simulink model "BiT_Template_V4"  (R2025b)
settings: Solver=FixedStepAuto  StartTime=0.0  StopTime=90  FixedStep=0.005  RelTol=1e-3
StopFcn:
  | user_confirmed = true;
  | disp('Gestoppt?!')
  | 
  | % stop(t);
  | % delete(t);
  | 
  | %% Switch to Config Mode
  | %Tc3_AI.sysManager.ActivateConfiguration();
  | %
  | % Tc3_AI.SwitchToConfig('local')
  | %
  | % %save Solution
  | % Tc3_AI.SaveSolution();
  | %
  | % %% Close Aktive VS Instance
  | % Tc3_AI.closeVsInstance();
libraries: simulink x1, slpidlib x1
settings Model: SimulationMode=external  Creator=clemensm  LastModifiedBy=Felix
settings OptimizationCC: LocalBlockOutputs=off
settings RTWCC: SystemTargetFile=TwinCatGrt.tlc  GenCodeOnly=on  GenerateMakefile=off  TemplateMakefile=tcgrt_msbuild.tmf  TargetLang=C++  Description=TwinCAT GRT Target
settings STFCustomTargetCC: SystemTargetFile=TwinCatGrt.tlc  TargetLangStandard=C++11 (ISO)  CombineOutputUpdateFcns=on  CodeInterfacePackaging=Reusable function  CPPClassGenCompliant=on  GRTInterface=off  GenerateAllocFcn=on  TcCom_OnlineChange=off  TcProject_PublishTcRTx64=on  TcProject_PublishConfiguration=Release  TcProject_CppLanguageStandard=Default  TcProject_Description=TwinCAT executable file, generated by TwinCAT $<ModuleGenerator:ProductId>  TcCom_GroupName=TE140x|Simulink Modules  TcProject_DataExchangeModulesVersion=$<ModuleGenerator:DataExchange:Version>  TcCom_BlockDiagramDebugInfoExport=on  TcCom_OutputDataAccess=Output Source DataArea  TcCom_OutputCreateSymbols=on  TcProject_LibraryCategories=$<VendorName>  TcCom_DWorkCreateSymbols=on  TcProject_UseStaticStlString=off  TcProject_PlcVarPrefixes=PVOID=p | BOOL=b | BOOL32=b | DATE=d | TIME_OF_DATE=td | TIME=t | LTIME=t | GUID=n  TcCom_UpdateExceptionHandling=CallerExceptions  TcCom_VariableSymbolMapping=Identical  TcProject_Publish=on  TcCom_BlockIoReadOnly=on  TcProject_VendorName=TE140x Module Vendor  TcCom_InputInitValues=off  TcCom_InputDataAccess=Input Destination DataArea  TcProject_LowestCompatibleTcBuild=$<TwinCAT:Version:BUILD>  TcProject_SignTwinCatCertName=MCI_2024_OEM.tccert  TcCom_StepSizeAdaptation=RequireMatchingTaskCycleTime  TcCom_OemLicenses=$<Project:OemLicenses>  TcCom_ExecutionSequence=UpdateBeforeOutputMapping  TcCom_OriginalIoBlockNames=off  TcProject_BuildWithWdk=inherit default  TcProject_GeneratePlcLibrary=off  TcProject_ForceRebuildForPublish=off  TcCom_CallerVerification=Default  TcProject_PublishTcRTx86=on  TcCom_TcComWrapperFbProperties=off  TcProject_StaticStlStringCapacity=Auto  TcCom_StrictAccessLock=on  TcProject_PublishTcOSARMv8A=off  TcProject_UseIntrinsics=on  TcProject_DrvProductVersion=$<DrvFileVersion>  TcProject_IncrementVersion=Revision  TcProject_VendorIcon=$<TE140x:Icon>  TcProject_PreferIntOverLong=off  TcProject_ClassFactoryName=$<Project:Name>  TcCom_ExtModeRtAllowForParameterChange=on  TcProject_InstallPlcLibrary=off  TcCom_BlockDiagramVariableAccess=AssignToParent  TcCom_OnlineChangeRestoreDataAreas=off  TcProject_UseTmxExtension=Auto  TcCom_ModuleCaller=CyclicTask  TcCom_InputReadOnly=off  TcCom_DWorkReadOnly=on  TcCom_BlockDiagramExport=on  TcProject_PublishTcOSx64=off  TcCom_ExtendSignalResolution=on  TcPlcFb_Generate=off  TcPlcFb_ExtModeRtAllowForParameterChange=off  TcProject_PublishPlatformtoolset=Auto  TcCom_ParametersCreateSymbols=on  TcProject_UseDataExchangeModules=off  TcProject_CreateScopedEnums=Auto  TcCom_GlobalParamDefaultSharing=Define  TcCom_ContStateCreateSymbols=on  TcPlcFb_MonitorExecutionTime=off  TcProject_UseCodeInfoExporter=on  TcCom_GroupDisplayName=$<GroupName>  TcCom_Generate=on  TcCom_InitExceptionHandling=CallerExceptions  TcProject_Copyright=Copyright $<VendorName> $<LocalDateTime:%Y>  TcCom_ResolveMaskedSubsystems=on  TcCom_ExtModeRtAllowExecutionCommands=on  TcPlcFb_ExtModeRtAllowExecutionCommands=off  TcProject_PublishTcOSARMv7A=off  TcCom_BlockIoDataAccess=Internal DataArea  TcProject_SignWithTwinCatCertificate=inherit default  TcCom_TcComWrapperFb=off  TcCom_OutputReadOnly=on  TcCom_AccessLockState=Auto  TcProject_DeployRestart=off  TcProject_UseCodeDescriptor=on  TcProject_EnableNewPlatforms=off  TcCom_Legacy_ModuleBuildInfoParam=on  TcCom_ModuleIcon=$<TE140x:Icon>  TcPlcFb_OemLicenses=$<Project:OemLicenses>  TcCom_InputCreateSymbols=on  TcProject_PreferToolArchitectureX64=on  TcProject_DrvFileVersion=$<VersionFromFile>  TcCom_MonitorExecutionTime=off  TcCom_ContStateDataAccess=Internal DataArea  TcCom_ContStateReadOnly=on  TcProject_GenerateStructDutsWithDefaultValues=Auto  TcProject_LibCatPath=$<Project:Dir>\$<Project:Name>.libcat.xml  TcCom_TcComWrapperFbPropertyMonitoring=NoMonitoring  TcProject_CLanguageStandard=Default  TcCom_ExtModeRtWaitForStart=off  TcProject_PublishParallel=on  TcProject_PublishTcUMx86=off  TcProject_UseNativeBlockDiagramExport=off  TcPlcFb_UpdateExceptionHandling=CallerExceptions  TcCom_DataStoreReadOnly=off  TcPlcFb_ExtModeRtWaitForStart=off  TcCom_GroupIcon=$<TE140x:Icon>  TcProject_PublishTcUMx64=off  TcProject_VersionSrc=$<LatestTMFile>  TcCom_ExecutionInfoOutput=off  TcCom_ExecutionInfoParam=on  TcProject_ProjectDir=C:\TwinCAT\3.1\CustomConfig\Modules\Ctrl_only  TcProject_BuildSystem=Auto  TcCom_ParametersInitValues=on  TcCom_ParametersReadOnly=off  TcCom_ParametersDataAccess=Internal DataArea  TcProject_MaxVisibleArrayElements=200U  TcProject_PublishTcOSARMv7M=off  TcCom_ExecuteModelCode=on  TcCom_DWorkDataAccess=Internal DataArea  TcProject_CoderCppNamespace=coder  TcProject_Generate=on  TcProject_Versioning=Versioned  TcProject_GenerateVsSolution=No  TcProject_Verbosity=Normal  TcProject_CreateUniqueEnumItemNames=off  TcCom_DataStoreDataAccess=None  TcCom_AllowDataAreaForSharedData=off  TcProject_ProductName=$<ModuleGenerator:ProductId> $<ModuleGenerator:Version:MAJOR.MINOR>  TcCom_DataStoreCreateSymbols=on  TcProject_UseDescriptorCodeType=on  TcPlcFb_InitExceptionHandling=CallerExceptions  TcProject_TmxInstall=on  TcCom_BlockIoCreateSymbols=on
settings GRTTargetCC: ExtMode=on  ExtModeMexFile=TcExtModeClient  MultiInstanceErrorCode=None  TargetLangStandard=C++11 (ISO)  ParMdlRefBuildCompliant=off  CompOptLevelCompliant=off  MatFileLogging=off  CodeInterfacePackaging=Reusable function  GenerateAllocFcn=on  UseToolchainInfoCompliant=off

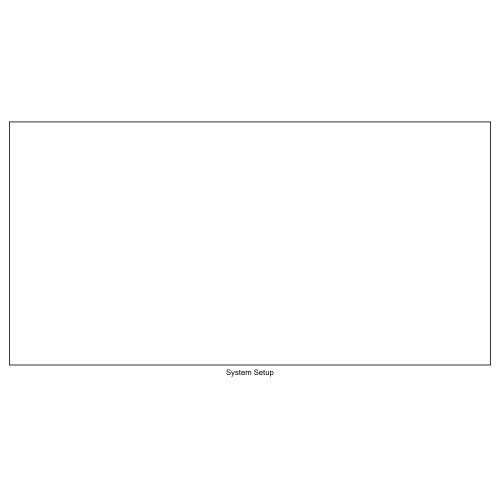
[thumbnail: Simulink's stored preview of the top-level diagram]
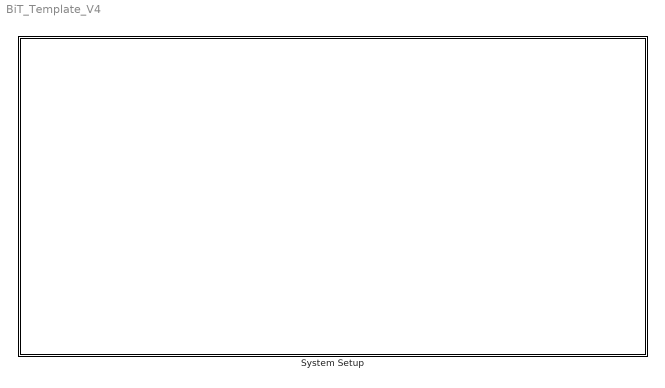
== system BiT_Template_V4 ==
  System Setup : Subsystem

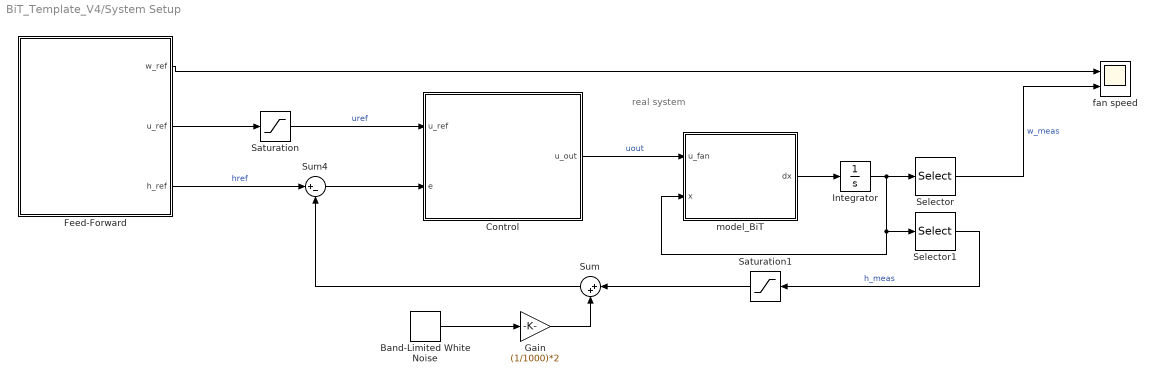
== system BiT_Template_V4/System Setup ==
  note: real system
  Band-Limited White Noise : simulink/Sources/Band-Limited White Noise  Cov=[0.9]  Ts=0.1  seed=[23341]
  Control : Subsystem
  Feed-Forward : Subsystem
  Gain : Gain  Gain=(1/1000)*2
  Integrator : Integrator  InitialCondition=[0.1;0;4200]  UpperSaturationLimit=[0.5;5;8000]  LowerSaturationLimit=0
  Saturation : Saturate  UpperLimit=100  LowerLimit=0
  Saturation1 : Saturate  LowerLimit=0
  Selector : Selector  InputPortWidth=3  IndexOptions=Index vector (dialog)  Indices=3  OutputSizes=1
  Selector1 : Selector  InputPortWidth=3  IndexOptions=Index vector (dialog)  Indices=1  OutputSizes=1
  Sum : Sum  Inputs=|++
  Sum4 : Sum  Inputs=|+-
  fan speed : Scope  NumInputPorts=2
      settings: TimeSpan=60  ActiveDisplayYMinimum=4192.4462547686062  ActiveDisplayYMaximum=4423.0615272479326
  model_BiT : MATLAB Function  TreatAsAtomicUnit=on
  wires:
  Selector/1 -> fan speed/2  "w_meas"
  Integrator/1 -> Selector/1, Selector1/1, model_BiT/2(x)
  Feed-Forward/1(w_ref) -> fan speed/1
  Sum4/1 -> Control/2(e)
  Feed-Forward/2(u_ref) -> Saturation/1
  Feed-Forward/3(h_ref) -> Sum4/1  "href"
  Saturation/1 -> Control/1(u_ref)  "uref"
  Band-Limited White Noise/1 -> Gain/1
  Control/1(u_out) -> model_BiT/1(u_fan)  "uout"
  model_BiT/1(dx) -> Integrator/1
  Selector1/1 -> Saturation1/1  "h_meas"
  Sum/1 -> Sum4/2
  Gain/1 -> Sum/2
  Saturation1/1 -> Sum/1

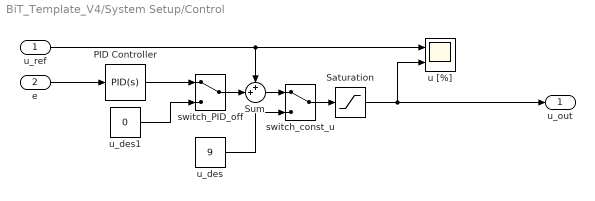
== system BiT_Template_V4/System Setup/Control ==
  u_ref : Inport
  e : Inport  Port=2
  PID Controller : slpidlib/PID Controller  Controller=PID  Form=Parallel  TimeDomain=Continuous-time  UseExternalTs=off  SampleTime=-1  IntegratorMethod=Forward Euler  FilterMethod=Forward Euler  ControllerParametersSource=internal  P=1  I=0.1  UseKiTs=off  D=1  UseExternalDerivativeSource=off  N=100  UseFilter=on  TunerSelectOption=Transfer Function Based (PID Tuner App)  InitialConditionSource=internal  InitialConditionForIntegrator=0  InitialConditionForFilter=0  DifferentiatorICPrevScaledInput=0  ExternalReset=none  TrackingMode=off  Kt=1  LimitOutput=off  SatLimitsSource=internal  UpperSaturationLimit=inf  LowerSaturationLimit=-inf  LinearizeAsGain=on  AntiWindupMode=none  Kb=1  LimitIntegrator=off  UpperIntegratorSaturationLimit=inf  LowerIntegratorSaturationLimit=-inf  POutMin=[]  POutMax=[]  IOutMin=[]  IOutMax=[]  DOutMin=[]  DOutMax=[]  NOutMin=[]  NOutMax=[]  SumOutMin=[]  SumOutMax=[]  SaturationOutMin=[]  SaturationOutMax=[]  PParamMin=[]  PParamMax=[]  IParamMin=[]  IParamMax=[]  DParamMin=[]  DParamMax=[]  NParamMin=[]  NParamMax=[]  KbParamMin=[]  KbParamMax=[]  KtParamMin=[]  KtParamMax=[]  KbOutMin=[]  KbOutMax=[]  KtOutMin=[]  KtOutMax=[]  IntegratorOutMin=[]  IntegratorOutMax=[]  FilterOutMin=[]  FilterOutMax=[]  SumI1OutMin=[]  SumI1OutMax=[]  SumI2OutMin=[]  SumI2OutMax=[]  SumI3OutMin=[]  SumI3OutMax=[]  SumI4OutMin=[]  SumI4OutMax=[]  SumDOutMin=[]  SumDOutMax=[]  DifferentiatorOutMin=[]  DifferentiatorOutMax=[]  FilterDiffOutCoefMin=[]  FilterDiffOutCoefMax=[]  ReciprocalOutMin=[]  ReciprocalOutMax=[]  SumDenOutMin=[]  SumDenOutMax=[]  SumNumOutMin=[]  SumNumOutMax=[]  DivideOutMin=[]  DivideOutMax=[]  UdiffTsProdOutMin=[]  UdiffTsProdOutMax=[]  NTsProdOutMin=[]  NTsProdOutMax=[]  UintegralTsProdOutMin=[]  UintegralTsProdOutMax=[]  UngainTsProdOutMin=[]  UngainTsProdOutMax=[]  ClampingZeroOutDataTypeStr=Inherit: Inherit via back propagation  ClampingZeroOutMin=[]  ClampingZeroOutMax=[]  FilterDenConstantOutDataTypeStr=Inherit: Inherit via back propagation  FilterDenConstantOutMin=[]  FilterDenConstantOutMax=[]  PCopyOutDataTypeStr=Inherit: Inherit via back propagation  PCopyOutMin=[]  PCopyOutMax=[]  NCopyOutDataTypeStr=Inherit: Inherit via back propagation  NCopyOutMin=[]  NCopyOutMax=[]  IntegratorContinuousStateAttributes=''  IntegratorStateMustResolveToSignalObject=off  IntegratorRTWStateStorageClass=Auto  FilterContinuousStateAttributes=''  FilterStateMustResolveToSignalObject=off  FilterRTWStateStorageClass=Auto  ParallelPVariant=InternalParameters  IdealPVariant=Disabled  IVariant=InternalParameters  DVariant=InternalParameters  IntegratorVariant=Continuous  SatVariant=Disabled  AWVariant=Passthrough  PCopyVariant=Disabled  TRVariant=Disabled  FdbkBlocksVariant=Forward  IdealPFdbkVariant=Disabled  SatFdbkVariant=Disabled  DerivativeFilterVariant=ContFilter  NVariant=InternalParameters  NCopyVariant=Disabled  FilterICVariant=InternalICsFilter  IntegratorICVariant=InternalICs  ExternalResetVariant=Disabled  TRSumVariant=Passthrough  SumFdbkVariant=Disabled  SumVariant=Sum_PID  TsampFilterVariant=InternalTs  TsampNgainVariant=Passthrough  TsampIntegralVariant=Disabled_SignalSpec  ExternalSaturationOutDataTypeStr=Inherit: Same as second input  DerivativeSourceVariant=ErrorSignal  PreIntVariant=InternalPreInt
  Saturation : Saturate  UpperLimit=100  LowerLimit=0
  Sum : Sum  Inputs=++|
  switch_PID_off : ManualSwitch
  switch_const_u : ManualSwitch
  u [%] : Scope  NumInputPorts=2
      settings: TimeSpan=60  ActiveDisplayYMinimum=7.1623782098242694  ActiveDisplayYMaximum=10.402299316136082
  u_des : Constant  Value=9
  u_des1 : Constant  Value=0
  u_out : Outport
  wires:
  e/1 -> PID Controller/1
  u_ref/1 -> u [%]/1, Sum/1
  Sum/1 -> switch_const_u/1
  PID Controller/1 -> switch_PID_off/1
  switch_PID_off/1 -> Sum/2
  u_des1/1 -> switch_PID_off/2
  Saturation/1 -> u_out/1, u [%]/2
  switch_const_u/1 -> Saturation/1
  u_des/1 -> switch_const_u/2

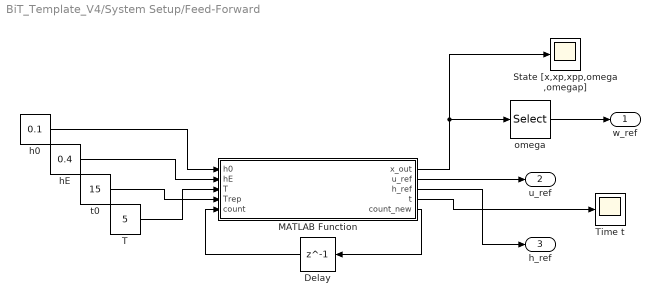
== system BiT_Template_V4/System Setup/Feed-Forward ==
  Delay : Delay  DelayLength=1
  MATLAB Function : MATLAB Function  TreatAsAtomicUnit=on
  State [x,xp,xpp,omega,omegap] : Scope
      settings: TimeSpan=60  ActiveDisplayYMinimum=-2.8507281834226665  ActiveDisplayYMaximum=4.5348179296068727
  T : Constant  Value=5
  Time t : Scope
      settings: ActiveDisplayYMinimum=-1  ActiveDisplayYMaximum=1
  h0 : Constant  Value=0.1
  hE : Constant  Value=0.4
  omega : Selector  InputPortWidth=5  IndexOptions=Index vector (dialog)  Indices=4  OutputSizes=1
  t0 : Constant  Value=15
  w_ref : Outport
  u_ref : Outport  Port=2
  h_ref : Outport  Port=3
  wires:
  h0/1 -> MATLAB Function/1(h0)
  MATLAB Function/4(t) -> Time t/1
  T/1 -> MATLAB Function/3(T)
  t0/1 -> MATLAB Function/4(Trep)
  Delay/1 -> MATLAB Function/5(count)
  MATLAB Function/5(count_new) -> Delay/1
  hE/1 -> MATLAB Function/2(hE)
  MATLAB Function/1(x_out) -> State [x,xp,xpp,omega,omegap]/1, omega/1
  MATLAB Function/2(u_ref) -> u_ref/1
  MATLAB Function/3(h_ref) -> h_ref/1
  omega/1 -> w_ref/1

== matlab function BiT_Template_V4/System Setup/model_BiT ==
  data: u_fan input; dx output; x input
function dx = model_BiT(u_fan, x)

alpha1 = 0.000745736;
alpha2 = 0.209195;
alpha3 = 9.81;
tau_omega = 1.255; 
u_0 = -34.234; 
k_omega = 96.295;

dx1 = x(2);
dx2 = (alpha1*x(3) - alpha2*x(2))^2 - alpha3;
dx3 = (k_omega*(u_fan-u_0)-x(3))/tau_omega;

dx = [dx1; dx2; dx3];
end

== matlab function BiT_Template_V4/System Setup/Feed-Forward/MATLAB Function ==
  data: x_out output; u_ref output; h_ref output; t output; h0 input; hE input; T input; Trep input; count input; count_new output
function [x_out,u_ref,h_ref,t,count_new] = feed_forward(h0,hE,T,Trep,count)

count_new = count+1;
dT = 0.005;
t = count_new*dT;

if mod(floor(t/Trep), 2)
    h0_traj = hE;
    hE_traj = h0;
else
    h0_traj = h0;
    hE_traj = hE;
end
    
alpha1 = 0.000745736;
alpha2 = 0.209195;
alpha3 = 9.81;
tau_omega = 1.255; 
u_0 = -34.234; 
k_omega = 96.295;

% Calculate Trajectory
x_ref = 0;
xp_ref = 0;
xpp_ref = 0;
xppp_ref = 0;


tau = rem(t, Trep);

if tau > T
    x_ref = hE_traj;
else
    a0 = h0_traj;
    a1 = 0;
    a2 = 0;
    a3 = 10*(hE_traj-h0_traj)/T^3;
    a4 = -15*(hE_traj-h0_traj)/T^4;
    a5 = 6*(hE_traj-h0_traj)/T^5;
    x_ref = a0 + a1*tau + a2*tau^2 + a3*tau^3 + a4*tau^4 + a5*tau^5;
    xp_ref = 3*a3*tau^2 + 4*a4*tau^3 + 5*a5*tau^4;
    xpp_ref = 6*a3*tau + 12*a4*tau^2 + 20*a5*tau^3;
    xppp_ref = 6*a3 + 24*a4*tau + 60*a5*tau^2;
    % Trajectory has to be implemented!
end

% Equations:
omega = (sqrt(xpp_ref + alpha3) + alpha2*xp_ref) / alpha1; % equation for omega
omega_p = ((xppp_ref / (2*sqrt(xpp_ref+alpha3)))+alpha2*xpp_ref) / alpha1; % equation for omega dot
u = (tau_omega * omega_p + omega)/k_omega + u_0; % equation for u
% yallah habibi
h_ref = x_ref;
u_ref = u; 
x_out = [x_ref,xp_ref,xpp_ref,omega,omega_p]';
end
